simulink model "untitled"  (R2016a)
settings: Solver=FixedStepDiscrete  StartTime=0.0  StopTime=100.0  FixedStep=0.01  RelTol=1e-3
settings Model: DataDictionary=new.sldd  Creator=91968  LastModifiedBy=91968

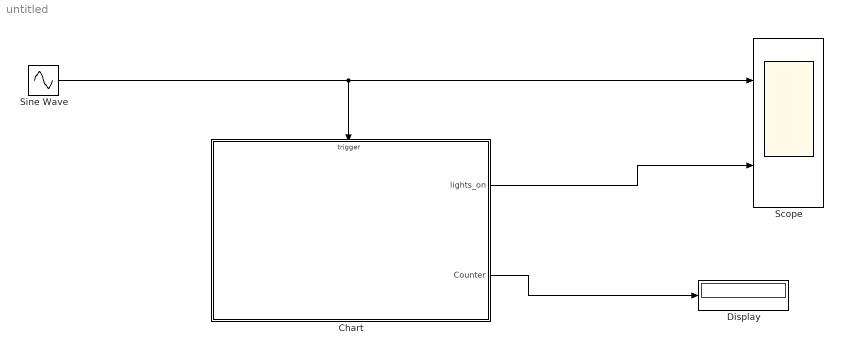
== system untitled ==
  Chart : Stateflow chart  TreatAsAtomicUnit=on
  Display : Display
  Scope : Scope  NumInputPorts=2
  Sine Wave : Sin  Frequency=0.62831  SampleTime=0
  wires:
  Sine Wave/1 -> Chart/Trigger, Scope/1
  Chart/2(Counter) -> Display/1
  Chart/1(lights_on) -> Scope/2

== stateflow chart untitled/Chart ==
  state Power_on
    entry:
    lights_on = 1;
  state Power_off
    entry:
    lights_on = 0;
  Power_off -> Power_on : Switch{Counter=Counter+1;}
  (default) -> Power_off
  Power_on -> Power_off : Switch{Counter=Counter+1;}
  data: lights_on output double =0; Counter output double =0
  events: Switch input RISING_EDGE_EVENT
